simulink model "example_simulink_DistanceSensor"  (Simulink 7.0)
settings: Solver=FixedStepDiscrete  StartTime=0.0  StopTime=inf  FixedStep=20  RelTol=1e-3
libraries: lib_robotinohardware x12
settings Model: Creator=indorewala  LastModifiedBy=indorewala

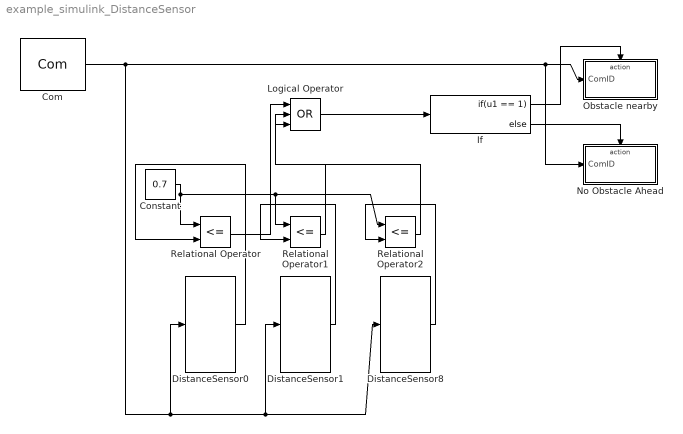
== system example_simulink_DistanceSensor ==
  Com : lib_robotinohardware/Com  ip='127.0.0.1'
  Constant : Constant  Value=0.7  OutDataType=sfix(16)  OutScaling=2^0
  DistanceSensor0 : lib_robotinohardware/DistanceSensor  num=0
  DistanceSensor1 : lib_robotinohardware/DistanceSensor  num=1
  DistanceSensor8 : lib_robotinohardware/DistanceSensor  num=8
  If : If  IfExpression=u1 == 1
  Logical Operator : Logic  Operator=OR  Inputs=3  AllPortsSameDT=off  OutDataTypeMode=boolean
  No Obstacle Ahead : Subsystem  TreatAsAtomicUnit=on
  Obstacle nearby : Subsystem  TreatAsAtomicUnit=on
  Relational Operator : RelationalOperator  Operator=<=  LogicOutDataTypeMode=boolean
  Relational Operator1 : RelationalOperator  Operator=<=  LogicOutDataTypeMode=boolean
  Relational Operator2 : RelationalOperator  Operator=<=  LogicOutDataTypeMode=boolean
  wires:
  Com/1 -> DistanceSensor0/1, DistanceSensor1/1, DistanceSensor8/1, Obstacle nearby/1(ComID), No Obstacle Ahead/1(ComID)
  Constant/1 -> Relational Operator/1, Relational Operator1/1, Relational Operator2/1
  DistanceSensor0/1 -> Relational Operator/2
  DistanceSensor1/1 -> Relational Operator1/2
  DistanceSensor8/1 -> Relational Operator2/2
  Relational Operator/1 -> Logical Operator/1
  Relational Operator1/1 -> Logical Operator/2
  Relational Operator2/1 -> Logical Operator/3
  Logical Operator/1 -> If/1
  If/2 -> No Obstacle Ahead/Action
  If/1 -> Obstacle nearby/Action

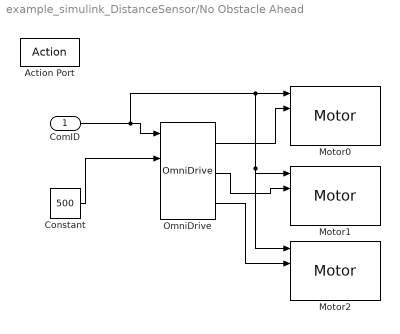
== system example_simulink_DistanceSensor/No Obstacle Ahead ==
  ComID : Inport  OutDataType=sfix(16)  OutScaling=2^0
  Action Port : ActionPort  ActionType=else
  Constant : Constant  Value=500  OutDataType=sfix(16)  OutScaling=2^0
  Motor0 : lib_robotinohardware/Motor  num=0  kp=0.9  ki=0.1  kd=0
  Motor1 : lib_robotinohardware/Motor  num=1  kp=0.9  ki=0.1  kd=0
  Motor2 : lib_robotinohardware/Motor  num=2  kp=0.9  ki=0.1  kd=0
  OmniDrive : lib_robotinohardware/OmniDrive
  wires:
  ComID/1 -> OmniDrive/1, Motor0/1, Motor2/1, Motor1/1
  Constant/1 -> OmniDrive/2
  OmniDrive/1 -> Motor0/2
  OmniDrive/2 -> Motor1/2
  OmniDrive/3 -> Motor2/2

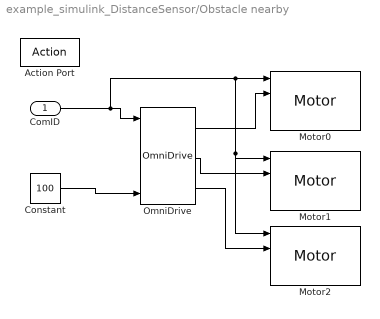
== system example_simulink_DistanceSensor/Obstacle nearby ==
  ComID : Inport  OutDataType=sfix(16)  OutScaling=2^0
  Action Port : ActionPort  ActionType=then
  Constant : Constant  Value=100  OutDataType=sfix(16)  OutScaling=2^0
  Motor0 : lib_robotinohardware/Motor  num=0  kp=0.9  ki=0.1  kd=0
  Motor1 : lib_robotinohardware/Motor  num=1  kp=0.9  ki=0.1  kd=0
  Motor2 : lib_robotinohardware/Motor  num=2  kp=0.9  ki=0.1  kd=0
  OmniDrive : lib_robotinohardware/OmniDrive
  wires:
  ComID/1 -> OmniDrive/1, Motor0/1, Motor1/1, Motor2/1
  Constant/1 -> OmniDrive/4
  OmniDrive/1 -> Motor0/2
  OmniDrive/2 -> Motor1/2
  OmniDrive/3 -> Motor2/2
